simulink model "gm_sampleModel1583_sub"  (R2023a)
settings: Solver=VariableStepAuto  StartTime=0.0  StopTime=10.0  RelTol=1e-3
libraries: simulink x1, hdlsllib x1
settings Model: Creator=user1  LastModifiedBy=user1
settings OptimizationCC: BlockReduction=off  ConditionallyExecuteInputs=off
settings DebuggingCC: InheritedTsInSrcMsg=none

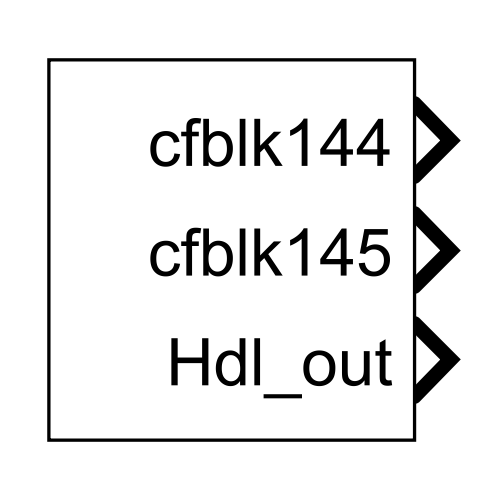
[thumbnail: Simulink's stored preview of the top-level diagram]
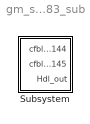
== system gm_sampleModel1583_sub ==
  Subsystem : Subsystem

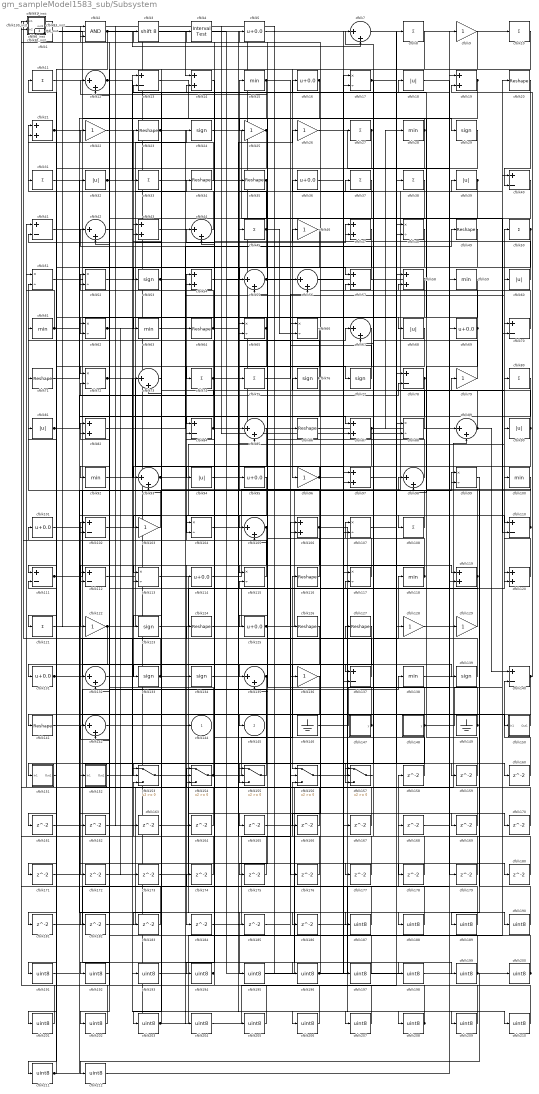
== system gm_sampleModel1583_sub/Subsystem ==
  cfblk1 : simulink/Logic and Bit Operations/Bit Set  iBit=0
      settings: LibrarySourceBlock=|
      | hdlsllib/Logic and Bit
      | Operations/Bit Set
  cfblk{8,10..11,27,31,33,37..38,45,50,74..75,80,108,121} (15 alike) : Sum  Inputs=+  OutDataTypeStr=uint8
  cfblk{15,28,59,61,63,92,100,118,138} (9 alike) : MinMax  OutDataTypeStr=uint8
  cfblk{5,16,36,69,95,101,114,125,131} (9 alike) : Bias  Bias=0.0  SaturateOnIntegerOverflow=off
  cfblk{13,40..41,70,78,84,102,110..112,137,140} (12 alike) : Sum  Inputs=+-  OutDataTypeStr=uint8
  cfblk{9,22,25..26,46,79,96,103,122,128..129,136} (12 alike) : Gain  OutDataTypeStr=uint8
  cfblk{17,48,51..52,62,65..66,72,88,99,104,107,113,115,117} (15 alike) : Product  Inputs=*/  OutDataTypeStr=uint8  RndMeth=Zero  SaturateOnIntegerOverflow=on
  cfblk{7,12,42,44,55..56,67,73,85,89,93,98,105,132,135,142} (16 alike) : Sum  Inputs=|++  OutDataTypeStr=uint8
  cfblk{14,19,21,43,47,54,57..58,82,87,97,106,119..120} (14 alike) : Sum  OutDataTypeStr=uint8
  cfblk109_inst : Subsystem
  cfblk{20,23,34..35,49,64,71,86,116,124,126..127,141} (13 alike) : Reshape
  cfblk{24,29,53,76..77,123,133..134,139} (9 alike) : Signum
  cfblk130_inst : Subsystem
  cfblk146 : Ground
  cfblk147 : Subsystem  mask(Counter Free-Running){NumBits=double(16), tsamp=double(-1)}
      mask prompts: NumBits "Simulink:masks:NumberOfBits_MP"; tsamp "Simulink:masks:SampleTime_MP"
      mask help: Simulink:masks:CounterFreeRunning_MD
  cfblk148 : Subsystem  mask(Counter Free-Running){NumBits=double(16), tsamp=double(-1)}
      mask prompts: NumBits "Simulink:masks:NumberOfBits_MP"; tsamp "Simulink:masks:SampleTime_MP"
      mask help: Simulink:masks:CounterFreeRunning_MD
  cfblk149 : Ground
  cfblk150 : Subsystem
  cfblk151 : Subsystem
  cfblk152 : Subsystem
  cfblk{153..157} (5 alike) : Switch  OutDataTypeStr=uint8  SaturateOnIntegerOverflow=off  InputSameDT=off
  cfblk{158..186} (29 alike) : Delay  SampleTime=1
  cfblk{18,32,39,60,68,81,90,94} (8 alike) : Abs  OutDataTypeStr=uint8  SaturateOnIntegerOverflow=off
  cfblk{187..212} (26 alike) : DataTypeConversion  OutDataTypeStr=uint8  SaturateOnIntegerOverflow=off  RndMeth=Floor
  cfblk2 : Logic  AllPortsSameDT=off  OutDataTypeStr=boolean
  cfblk3 : ArithShift  BitShiftNumber=8
  cfblk30_inst : Subsystem
  cfblk4 : hdlsllib/Logic and Bit Operations/Interval Test  IntervalClosedRight=on  uplimit=0.5  IntervalClosedLeft=on  lowlimit=-0.5  OutDataTypeStr=uint8
  cfblk6_inst : Subsystem
  cfblk83_inst : Subsystem
  cfblk91_inst : Subsystem
  cfblk144 : Outport  OutDataTypeStr=uint8  SampleTime=1  VectorParamsAs1DForOutWhenUnconnected=off
  cfblk145 : Outport  Port=2  OutDataTypeStr=uint8  SampleTime=1  VectorParamsAs1DForOutWhenUnconnected=off
  Hdl_out : Outport  Port=3  OutDataTypeStr=uint8  SampleTime=1
  wires:
  cfblk1/1 -> cfblk199/1
  cfblk10/1 -> cfblk96/1
  cfblk100/1 -> cfblk15/1
  cfblk101/1 -> cfblk135/1
  cfblk102/1 -> cfblk47/1
  cfblk103/1 -> cfblk51/2
  cfblk104/1 -> cfblk108/1
  cfblk105/1 -> cfblk54/1, cfblk172/1
  cfblk106/1 -> cfblk41/2, cfblk209/1, cfblk184/1
  cfblk107/1 -> cfblk79/1
  cfblk108/1 -> cfblk71/1
  cfblk109_inst/1(out1) -> cfblk10/1
  cfblk11/1 -> cfblk29/1
  cfblk110/1 -> cfblk13/2, cfblk50/1
  cfblk111/1 -> cfblk95/1, cfblk155/3
  cfblk112/1 -> cfblk34/1
  cfblk113/1 -> cfblk165/1
  cfblk114/1 -> cfblk17/2
  cfblk115/1 -> cfblk83_inst/1(in1)
  cfblk116/1 -> cfblk3/1
  cfblk117/1 -> cfblk46/1
  cfblk118/1 -> cfblk12/1, cfblk115/1, cfblk107/1
  cfblk119/1 -> cfblk76/1, cfblk115/2
  cfblk12/1 -> cfblk57/1, cfblk177/1
  cfblk120/1 -> cfblk70/1
  cfblk121/1 -> cfblk102/1
  cfblk122/1 -> cfblk24/1, cfblk131/1
  cfblk123/1 -> cfblk117/2
  cfblk124/1 -> cfblk100/1
  cfblk125/1 -> cfblk39/1, cfblk45/1
  cfblk126/1 -> cfblk161/1
  cfblk127/1 -> cfblk156/1
  cfblk128/1 -> cfblk69/1
  cfblk129/1 -> cfblk22/1
  cfblk13/1 -> cfblk85/2
  cfblk130_inst/1(out1) -> cfblk89/1, cfblk88/2, cfblk122/1
  cfblk131/1 -> cfblk153/2, cfblk118/1
  cfblk132/1 -> cfblk23/1
  cfblk133/1 -> cfblk6_inst/2(in2), cfblk169/1
  cfblk134/1 -> cfblk67/1
  cfblk135/1 -> cfblk181/1, cfblk75/1
  cfblk136/1 -> cfblk192/1
  cfblk137/1 -> cfblk5/1
  cfblk138/1 -> cfblk120/1
  cfblk139/1 -> cfblk7/1
  cfblk14/1 -> cfblk114/1
  cfblk140/1 -> cfblk19/2, cfblk141/1
  cfblk141/1 -> cfblk138/1
  cfblk142/1 -> cfblk160/1
  cfblk146/1 -> cfblk9/1
  cfblk147/1(y) -> cfblk116/1, cfblk65/2
  cfblk148/1(y) -> cfblk70/2, cfblk65/1, cfblk151/1(In1)
  cfblk149/1 -> cfblk67/2, cfblk101/1
  cfblk15/1 -> cfblk56/1, cfblk162/1
  cfblk150/1(Out1) -> cfblk145/1
  cfblk151/1(Out1) -> cfblk61/1
  cfblk152/1(Out1) -> cfblk124/1
  cfblk153/1 -> cfblk195/1
  cfblk154/1 -> cfblk42/2, cfblk126/1
  cfblk155/1 -> cfblk82/1
  cfblk156/1 -> cfblk48/1
  cfblk157/1 -> cfblk37/1
  cfblk158/1 -> cfblk44/1
  cfblk159/1 -> cfblk98/1
  cfblk16/1 -> cfblk123/1, cfblk112/1, cfblk105/2, cfblk104/2, cfblk74/1
  cfblk160/1 -> cfblk140/2
  cfblk161/1 -> cfblk154/1
  cfblk162/1 -> cfblk48/2
  cfblk163/1 -> cfblk89/2
  cfblk164/1 -> cfblk51/1
  cfblk165/1 -> cfblk198/1
  cfblk166/1 -> cfblk130_inst/2(in2)
  cfblk167/1 -> cfblk17/1
  cfblk168/1 -> cfblk120/2
  cfblk169/1 -> cfblk132/2
  cfblk17/1 -> cfblk78/1, cfblk157/3
  cfblk170/1 -> cfblk84/2
  cfblk171/1 -> cfblk155/1
  cfblk172/1 -> cfblk157/2
  cfblk173/1 -> cfblk85/1
  cfblk174/1 -> cfblk6_inst/1(in1)
  cfblk175/1 -> cfblk153/3
  cfblk176/1 -> cfblk156/3
  cfblk177/1 -> cfblk82/2
  cfblk178/1 -> cfblk155/2
  cfblk179/1 -> cfblk47/2
  cfblk18/1 -> cfblk179/1
  cfblk180/1 -> cfblk111/2
  cfblk181/1 -> cfblk119/2
  cfblk182/1 -> cfblk87/2
  cfblk183/1 -> cfblk109_inst/1(in1)
  cfblk184/1 -> cfblk156/2
  cfblk185/1 -> cfblk106/1
  cfblk186/1 -> cfblk188/1
  cfblk187/1 -> cfblk81/1
  cfblk188/1 -> cfblk4/1
  cfblk189/1 -> cfblk158/1
  cfblk19/1 -> cfblk68/1, cfblk102/2
  cfblk190/1 -> cfblk99/1
  cfblk191/1 -> cfblk99/2
  cfblk192/1 -> cfblk142/1
  cfblk193/1 -> cfblk136/1
  cfblk194/1 -> cfblk64/1, cfblk154/3
  cfblk195/1 -> cfblk38/1
  cfblk196/1 -> cfblk97/1, cfblk16/1, cfblk168/1
  cfblk197/1 -> cfblk33/1
  cfblk198/1 -> cfblk1/1
  cfblk199/1 -> cfblk212/1, cfblk88/1
  cfblk2/1 -> cfblk7/2, cfblk191/1
  cfblk20/1 -> cfblk40/2
  cfblk200/1 -> cfblk44/2, cfblk142/2
  cfblk201/1 -> cfblk91_inst/1(in1)
  cfblk202/1 -> cfblk91_inst/2(in2)
  cfblk203/1 -> cfblk20/1, cfblk113/2
  cfblk204/1 -> cfblk8/1
  cfblk205/1 -> cfblk14/2
  cfblk206/1 -> cfblk30_inst/1(in1)
  cfblk207/1 -> cfblk30_inst/2(in2)
  cfblk208/1 -> cfblk52/1, cfblk174/1
  cfblk209/1 -> cfblk43/1
  cfblk21/1 -> cfblk180/1, cfblk150/1(In1)
  cfblk210/1 -> cfblk43/2
  cfblk211/1 -> cfblk127/1, cfblk11/1
  cfblk212/1 -> cfblk59/1
  cfblk22/1 -> cfblk193/1
  cfblk23/1 -> cfblk204/1, cfblk110/1
  cfblk24/1 -> cfblk110/2
  cfblk25/1 -> cfblk182/1, cfblk121/1
  cfblk26/1 -> cfblk129/1
  cfblk27/1 -> cfblk201/1, cfblk154/2
  cfblk28/1 -> cfblk73/2, cfblk106/2, cfblk25/1
  cfblk29/1 -> cfblk93/1
  cfblk3/1 -> cfblk14/1
  cfblk30_inst/1(out1) -> cfblk205/1
  cfblk31/1 -> cfblk53/1
  cfblk32/1 -> cfblk54/2, cfblk18/1, cfblk178/1
  cfblk33/1 -> cfblk196/1
  cfblk34/1 -> cfblk21/1
  cfblk35/1 -> cfblk55/1, cfblk62/2, cfblk175/1
  cfblk36/1 -> cfblk190/1
  cfblk37/1 -> cfblk84/1
  cfblk38/1 -> cfblk194/1
  cfblk39/1 -> cfblk55/2, cfblk137/1
  cfblk4/1 -> cfblk187/1
  cfblk40/1 -> cfblk133/1
  cfblk41/1 -> cfblk185/1
  cfblk42/1 -> cfblk139/1
  cfblk43/1 -> cfblk208/1
  cfblk44/1 -> cfblk2/1
  cfblk45/1 -> cfblk21/2, cfblk202/1, cfblk66/2
  cfblk46/1 -> cfblk134/1
  cfblk47/1 -> cfblk132/1
  cfblk48/1 -> cfblk111/1
  cfblk49/1 -> cfblk103/1
  cfblk5/1 -> cfblk167/1
  cfblk50/1 -> cfblk113/1, cfblk63/1
  cfblk51/1 -> cfblk128/1
  cfblk52/1 -> cfblk163/1
  cfblk53/1 -> cfblk206/1, cfblk107/2
  cfblk54/1 -> cfblk77/1
  cfblk55/1 -> cfblk105/1, cfblk170/1
  cfblk56/1 -> cfblk27/1
  cfblk57/1 -> cfblk42/1
  cfblk58/1 -> cfblk137/2, Hdl_out/1
  cfblk59/1 -> cfblk211/1
  cfblk6_inst/1(out1) -> cfblk35/1
  cfblk60/1 -> cfblk83_inst/2(in2)
  cfblk61/1 -> cfblk86/1, cfblk41/1
  cfblk62/1 -> cfblk210/1, cfblk173/1
  cfblk63/1 -> cfblk60/1
  cfblk64/1 -> cfblk40/1, cfblk2/2
  cfblk65/1 -> cfblk72/1, cfblk62/1
  cfblk66/1 -> cfblk171/1
  cfblk67/1 -> cfblk153/1
  cfblk68/1 -> cfblk125/1
  cfblk69/1 -> cfblk98/2, cfblk57/2
  cfblk7/1 -> cfblk159/1
  cfblk70/1 -> cfblk109_inst/2(in2)
  cfblk71/1 -> cfblk32/1
  cfblk72/1 -> cfblk176/1, cfblk117/1
  cfblk73/1 -> cfblk183/1
  cfblk74/1 -> cfblk12/2, cfblk72/2, cfblk26/1
  cfblk75/1 -> cfblk56/2
  cfblk76/1 -> cfblk112/2, cfblk31/1
  cfblk77/1 -> cfblk66/1
  cfblk78/1 -> cfblk157/1, cfblk152/1(In1)
  cfblk79/1 -> cfblk36/1
  cfblk8/1 -> cfblk203/1
  cfblk80/1 -> cfblk135/2
  cfblk81/1 -> cfblk78/2, cfblk186/1, cfblk104/1
  cfblk82/1 -> cfblk49/1
  cfblk83_inst/1(out1) -> cfblk164/1
  cfblk84/1 -> cfblk87/1, cfblk52/2
  cfblk85/1 -> cfblk93/2
  cfblk86/1 -> cfblk19/1
  cfblk87/1 -> cfblk97/2, cfblk28/1
  cfblk88/1 -> cfblk13/1
  cfblk89/1 -> cfblk58/2, cfblk140/1
  cfblk9/1 -> cfblk92/1
  cfblk90/1 -> cfblk58/1, cfblk166/1
  cfblk91_inst/1(out1) -> cfblk200/1
  cfblk92/1 -> cfblk73/1
  cfblk93/1 -> cfblk90/1, cfblk197/1
  cfblk94/1 -> cfblk207/1
  cfblk95/1 -> cfblk144/1
  cfblk96/1 -> cfblk94/1, cfblk119/1
  cfblk97/1 -> cfblk80/1
  cfblk98/1 -> cfblk130_inst/1(in1)
  cfblk99/1 -> cfblk189/1

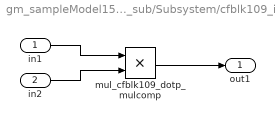
== system gm_sampleModel1583_sub/Subsystem/cfblk109_inst ==
  in1 : Inport  OutDataTypeStr=uint8  SampleTime=1
  in2 : Inport  Port=2  OutDataTypeStr=uint8  SampleTime=1
  mul_cfblk109_dotp_mulcomp : Product  Inputs=**  OutDataTypeStr=uint8  SampleTime=1
  out1 : Outport  OutDataTypeStr=uint8  SampleTime=1
  wires:
  in1/1 -> mul_cfblk109_dotp_mulcomp/1
  in2/1 -> mul_cfblk109_dotp_mulcomp/2
  mul_cfblk109_dotp_mulcomp/1 -> out1/1

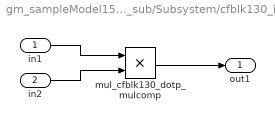
== system gm_sampleModel1583_sub/Subsystem/cfblk130_inst ==
  in1 : Inport  OutDataTypeStr=uint8  SampleTime=1
  in2 : Inport  Port=2  OutDataTypeStr=uint8  SampleTime=1
  mul_cfblk130_dotp_mulcomp : Product  Inputs=**  OutDataTypeStr=uint8  SampleTime=1
  out1 : Outport  OutDataTypeStr=uint8  SampleTime=1
  wires:
  in1/1 -> mul_cfblk130_dotp_mulcomp/1
  in2/1 -> mul_cfblk130_dotp_mulcomp/2
  mul_cfblk130_dotp_mulcomp/1 -> out1/1

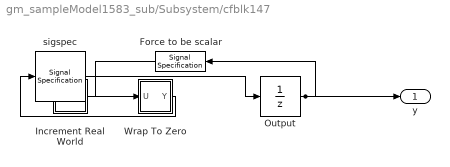
== system gm_sampleModel1583_sub/Subsystem/cfblk147 ==
  Force to be scalar : SignalSpecification  DisableCoverage=on  Dimensions=1
  Increment Real World : Subsystem  mask(Real World Value Increment){}
      mask help: Simulink:masks:RealWorldValueIncrement_MD
      mask Display: disp('V++')
  Output : UnitDelay  InitialCondition=0.0  SampleTime=tsamp  HasFrameUpgradeWarning=on
  Wrap To Zero : Subsystem  mask(Wrap To Zero){Threshold=double(65535)}
      mask prompts: Threshold "Simulink:masks:Threshold_MP"
      mask help: Simulink:masks:WrapToZero_MD
  sigspec : SignalSpecification  OutDataTypeStr=uint16  Dimensions=1
  y : Outport  SampleTime=1
  wires:
  Force to be scalar/1 -> Increment Real World/1(u)
  Increment Real World/1(y) -> Wrap To Zero/1(U)
  Output/1 -> Force to be scalar/1, y/1
  Wrap To Zero/1(Y) -> sigspec/1
  sigspec/1 -> Output/1

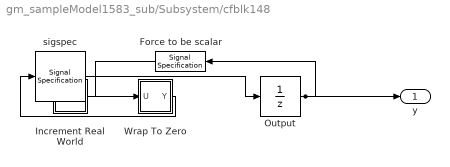
== system gm_sampleModel1583_sub/Subsystem/cfblk148 ==
  Force to be scalar : SignalSpecification  DisableCoverage=on  Dimensions=1
  Increment Real World : Subsystem  mask(Real World Value Increment){}
      mask help: Simulink:masks:RealWorldValueIncrement_MD
      mask Display: disp('V++')
  Output : UnitDelay  InitialCondition=0.0  SampleTime=tsamp  HasFrameUpgradeWarning=on
  Wrap To Zero : Subsystem  mask(Wrap To Zero){Threshold=double(65535)}
      mask prompts: Threshold "Simulink:masks:Threshold_MP"
      mask help: Simulink:masks:WrapToZero_MD
  sigspec : SignalSpecification  OutDataTypeStr=uint16  Dimensions=1
  y : Outport  SampleTime=1
  wires:
  Force to be scalar/1 -> Increment Real World/1(u)
  Increment Real World/1(y) -> Wrap To Zero/1(U)
  Output/1 -> Force to be scalar/1, y/1
  Wrap To Zero/1(Y) -> sigspec/1
  sigspec/1 -> Output/1

== system gm_sampleModel1583_sub/Subsystem/cfblk150 ==
  In1 : Inport  OutDataTypeStr=uint8  PortDimensions=1  SampleTime=1
  Out1 : Outport  SampleTime=1
  wires:
  In1/1 -> Out1/1

== system gm_sampleModel1583_sub/Subsystem/cfblk151 ==
  In1 : Inport  OutDataTypeStr=uint16  PortDimensions=1  SampleTime=1
  Out1 : Outport  SampleTime=1
  wires:
  In1/1 -> Out1/1

== system gm_sampleModel1583_sub/Subsystem/cfblk152 ==
  In1 : Inport  OutDataTypeStr=uint8  PortDimensions=1  SampleTime=1
  Out1 : Outport  SampleTime=1
  wires:
  In1/1 -> Out1/1

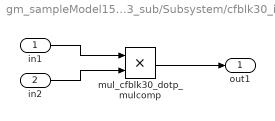
== system gm_sampleModel1583_sub/Subsystem/cfblk30_inst ==
  in1 : Inport  OutDataTypeStr=uint8  SampleTime=1
  in2 : Inport  Port=2  OutDataTypeStr=uint8  SampleTime=1
  mul_cfblk30_dotp_mulcomp : Product  Inputs=**  OutDataTypeStr=uint8  SampleTime=1
  out1 : Outport  OutDataTypeStr=uint8  SampleTime=1
  wires:
  in1/1 -> mul_cfblk30_dotp_mulcomp/1
  in2/1 -> mul_cfblk30_dotp_mulcomp/2
  mul_cfblk30_dotp_mulcomp/1 -> out1/1

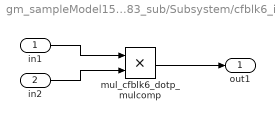
== system gm_sampleModel1583_sub/Subsystem/cfblk6_inst ==
  in1 : Inport  OutDataTypeStr=uint8  SampleTime=1
  in2 : Inport  Port=2  OutDataTypeStr=uint8  SampleTime=1
  mul_cfblk6_dotp_mulcomp : Product  Inputs=**  OutDataTypeStr=uint8  SampleTime=1
  out1 : Outport  OutDataTypeStr=uint8  SampleTime=1
  wires:
  in1/1 -> mul_cfblk6_dotp_mulcomp/1
  in2/1 -> mul_cfblk6_dotp_mulcomp/2
  mul_cfblk6_dotp_mulcomp/1 -> out1/1

== system gm_sampleModel1583_sub/Subsystem/cfblk83_inst ==
  in1 : Inport  OutDataTypeStr=uint8  SampleTime=1
  in2 : Inport  Port=2  OutDataTypeStr=uint8  SampleTime=1
  mul_cfblk83_dotp_mulcomp : Product  Inputs=**  OutDataTypeStr=uint8  SampleTime=1
  out1 : Outport  OutDataTypeStr=uint8  SampleTime=1
  wires:
  in1/1 -> mul_cfblk83_dotp_mulcomp/1
  in2/1 -> mul_cfblk83_dotp_mulcomp/2
  mul_cfblk83_dotp_mulcomp/1 -> out1/1

== system gm_sampleModel1583_sub/Subsystem/cfblk91_inst ==
  in1 : Inport  OutDataTypeStr=uint8  SampleTime=1
  in2 : Inport  Port=2  OutDataTypeStr=uint8  SampleTime=1
  mul_cfblk91_dotp_mulcomp : Product  Inputs=**  OutDataTypeStr=uint8  SampleTime=1
  out1 : Outport  OutDataTypeStr=uint8  SampleTime=1
  wires:
  in1/1 -> mul_cfblk91_dotp_mulcomp/1
  in2/1 -> mul_cfblk91_dotp_mulcomp/2
  mul_cfblk91_dotp_mulcomp/1 -> out1/1

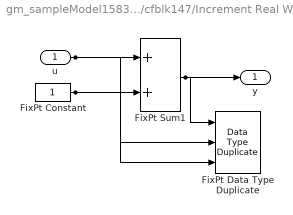
== system gm_sampleModel1583_sub/Subsystem/cfblk147/Increment Real World ==
  u : Inport  OutDataTypeStr=uint16  SampleTime=1
  FixPt Constant : Constant  DisableCoverage=on  OutDataTypeStr=Inherit: Inherit via back propagation  SampleTime=-1
  FixPt Data Type Duplicate : DataTypeDuplicate  DisableCoverage=on  NumInputPorts=3
  FixPt Sum1 : Sum  InputSameDT=on  OutDataTypeStr=Inherit: Inherit via back propagation  LockScale=on
  y : Outport  SampleTime=1
  wires:
  u/1 -> FixPt Sum1/1, FixPt Data Type Duplicate/2
  FixPt Constant/1 -> FixPt Sum1/2, FixPt Data Type Duplicate/3
  FixPt Sum1/1 -> FixPt Data Type Duplicate/1, y/1

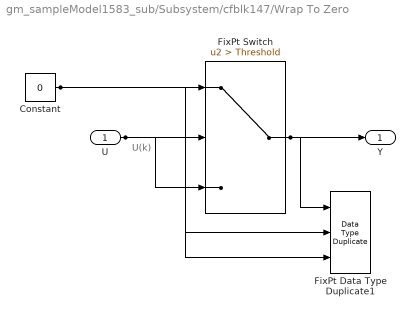
== system gm_sampleModel1583_sub/Subsystem/cfblk147/Wrap To Zero ==
  note: U(k)
  U : Inport  OutDataTypeStr=uint16  SampleTime=1
  Constant : Constant  DisableCoverage=on  Value=0  OutDataTypeStr=Inherit: Inherit via back propagation  SampleTime=-1
  FixPt Data Type Duplicate1 : DataTypeDuplicate  DisableCoverage=on  NumInputPorts=3
  FixPt Switch : Switch  Criteria=u2 > Threshold  Threshold=Threshold  OutDataTypeStr=Inherit: Inherit via back propagation  ZeroCross=off  SaturateOnIntegerOverflow=off  InputSameDT=off
  Y : Outport  SampleTime=1
  wires:
  U/1 -> FixPt Switch/3, FixPt Switch/2, FixPt Data Type Duplicate1/2
  Constant/1 -> FixPt Switch/1, FixPt Data Type Duplicate1/3
  FixPt Switch/1 -> FixPt Data Type Duplicate1/1, Y/1

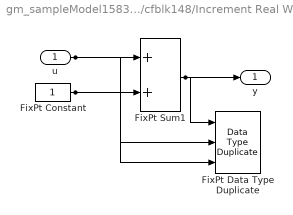
== system gm_sampleModel1583_sub/Subsystem/cfblk148/Increment Real World ==
  u : Inport  OutDataTypeStr=uint16  SampleTime=1
  FixPt Constant : Constant  DisableCoverage=on  OutDataTypeStr=Inherit: Inherit via back propagation  SampleTime=-1
  FixPt Data Type Duplicate : DataTypeDuplicate  DisableCoverage=on  NumInputPorts=3
  FixPt Sum1 : Sum  InputSameDT=on  OutDataTypeStr=Inherit: Inherit via back propagation  LockScale=on
  y : Outport  SampleTime=1
  wires:
  u/1 -> FixPt Sum1/1, FixPt Data Type Duplicate/2
  FixPt Constant/1 -> FixPt Sum1/2, FixPt Data Type Duplicate/3
  FixPt Sum1/1 -> FixPt Data Type Duplicate/1, y/1

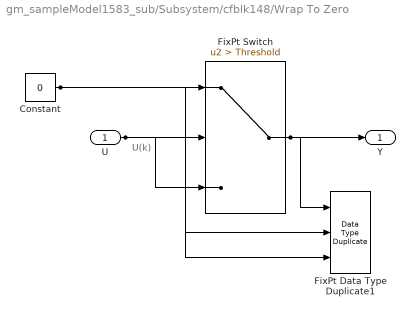
== system gm_sampleModel1583_sub/Subsystem/cfblk148/Wrap To Zero ==
  note: U(k)
  U : Inport  OutDataTypeStr=uint16  SampleTime=1
  Constant : Constant  DisableCoverage=on  Value=0  OutDataTypeStr=Inherit: Inherit via back propagation  SampleTime=-1
  FixPt Data Type Duplicate1 : DataTypeDuplicate  DisableCoverage=on  NumInputPorts=3
  FixPt Switch : Switch  Criteria=u2 > Threshold  Threshold=Threshold  OutDataTypeStr=Inherit: Inherit via back propagation  ZeroCross=off  SaturateOnIntegerOverflow=off  InputSameDT=off
  Y : Outport  SampleTime=1
  wires:
  U/1 -> FixPt Switch/3, FixPt Switch/2, FixPt Data Type Duplicate1/2
  Constant/1 -> FixPt Switch/1, FixPt Data Type Duplicate1/3
  FixPt Switch/1 -> FixPt Data Type Duplicate1/1, Y/1
